simulink model "PGA_MPC_MODEL"  (R2024b)
settings: Solver=ode4  StartTime=0.0  StopTime=180  FixedStep=0.0005  RelTol=1e-3
values from neighbouring files (symbols this model uses):
  Road_Curvature_Map = [Global_S, Global_K]    [Road_Condition_Info.m]
  Road_Mu_Map = [Global_S, Global_Mu]    [Road_Condition_Info.m]
  Target_Speed_Map = [Global_S, Global_Vx]    [Road_Condition_Info.m]
undefined symbols (not defined in the file or in its folder): MotorData, Sim_Mu_Set, Sim_Vx_Set
libraries: Solver_SF x1
(part 3 of 3)

== matlab function PGA_MPC_MODEL/Subsystem1/MATLAB Function ==
  data: x_curr input; T_final_opt output; Solver_Status output; x_ref input; T_ref_upper_in input size=[4 1]; Vehicle_State input; Stiffness_Input input size=[2 1]; NN_Weights input; Constraints input; dt_in input; Mu_in input; Curv_in input; Delta_f_in input; Debug_Info output size=[5 1]
function [T_final_opt, Solver_Status, Debug_Info] = Lower_Layer_MPC_Fixed(...
x_curr, x_ref, T_ref_upper_in, Vehicle_State, Stiffness_Input, ...
NN_Weights, Constraints,dt_in, Mu_in, Curv_in, Delta_f_in) 
%#codegen
% =========================================================================
% 下层 MPC v44.0 (纯净执行者版：剔除所有底层干预规则，100% 权力移交 AI)
% =========================================================================
%% 0. 强制初始化
T_final_opt = zeros(4, 1, 'double');
Solver_Status = 0.0;
Debug_Info = zeros(5, 1, 'double');

%% 1. 解析 Vehicle_State 与滤波
Veh_State = double(reshape(Vehicle_State, 6, 1)); 
Vx = max(Veh_State(1), 1.0); 
Fz_fl_raw = max(Veh_State(3), 1000.0); Fz_fr_raw = max(Veh_State(4), 1000.0);
Fz_rl_raw = max(Veh_State(5), 1000.0); Fz_rr_raw = max(Veh_State(6), 1000.0);
persistent u_prev is_initialized Fz_fl_f Fz_fr_f Fz_rl_f Fz_rr_f
if isempty(u_prev)
u_prev = zeros(4, 1); 
Fz_fl_f = Fz_fl_raw; Fz_fr_f = Fz_fr_raw;
Fz_rl_f = Fz_rl_raw; Fz_rr_f = Fz_rr_raw;
is_initialized = false; 
end
alpha_fz = 0.2; 
Fz_fl_f = (1 - alpha_fz) * Fz_fl_f + alpha_fz * Fz_fl_raw;
Fz_fr_f = (1 - alpha_fz) * Fz_fr_f + alpha_fz * Fz_fr_raw;
Fz_rl_f = (1 - alpha_fz) * Fz_rl_f + alpha_fz * Fz_rl_raw;
Fz_rr_f = (1 - alpha_fz) * Fz_rr_f + alpha_fz * Fz_rr_raw;
Fz_fl = Fz_fl_f; Fz_fr = Fz_fr_f; Fz_rl = Fz_rl_f; Fz_rr = Fz_rr_f;
Fz_total = Fz_fl + Fz_fr + Fz_rl + Fz_rr;
dt = double(dt_in(1)); if dt <= 0, dt = 0.01; end
beta_in = double(x_curr(1)); r_in = double(x_curr(2));
x_ref_safe = double(reshape(x_ref, 2, 1));
% ★ 增加低通滤波隔离上层可能的高频毛刺 ★
T_ref_upper_raw = double(reshape(T_ref_upper_in, 4, 1)); 
persistent T_ref_filtered
if isempty(T_ref_filtered), T_ref_filtered = zeros(4, 1); end
alpha_T = 0.15; 
T_ref_filtered = (1 - alpha_T) * T_ref_filtered + alpha_T * T_ref_upper_raw;
T_ref_upper = T_ref_filtered; 
T_total_req = sum(T_ref_upper); 
delta_f_rad = double(Delta_f_in(1)); 

%% 2. 计算危险度 (仅用于摩擦圆限幅，不再用于权重干预)
rho_real = abs(double(Curv_in(1))); 
if rho_real < 1e-4, rho_real = 1e-4; end
ay_req_feedforward = (Vx^2) * rho_real; 
mu_est = max(0.15, double(Mu_in(1))); 
ay_max = mu_est * 9.81;
kappa_dyn = min(ay_req_feedforward / ay_max, 0.98);

%% 3. 提取贝叶斯权重 (完全绝对信任 AI)
Weights = double(reshape(NN_Weights, 5, 1));
Q_beta = max(Weights(1), 10.0); 
Q_yaw = max(Weights(2), 10.0);
R_alloc = max(Weights(3), 1.0); 
R_rate_base = max(Weights(4), 10.0); 
R_rate_vec = R_rate_base * ones(4, 1); 
% 绝对执行 AI 给出的防滑权重！
W_slip_base = max(Weights(5), 0.1);
W_slip_vec = zeros(4, 1);
W_slip_vec(1) = W_slip_base * ((Fz_total / 4) / Fz_fl);
W_slip_vec(2) = W_slip_base * ((Fz_total / 4) / Fz_fr);
W_slip_vec(3) = W_slip_base * ((Fz_total / 4) / Fz_rl);
W_slip_vec(4) = W_slip_base * ((Fz_total / 4) / Fz_rr);
%% 4. 总转矩硬约束 (废除 Mode_Signal 的规则干预)
% ★ 强制写死为 500000，确保总需求不打折，底层再无借口！
W_sum = 20000.0; 
%% 5. 前角前馈 LTV 模型构建 
Cf = double(Stiffness_Input(1)); Cr = double(Stiffness_Input(2));
if Cf < 20000, Cf = Cf * 57.3; end; if Cr < 20000, Cr = Cr * 57.3; end
Np = 25; Nc = 2; nx = 2; nu = 4;
m = 1810; Iz = 2765; lf = 1.152; lr = 1.528;
Cr_safe = max(Cr, Cf * (lf / lr) * 0.85); 
a11 = -(Cf + Cr_safe) / (m * Vx); 
a12 = ((lr * Cr_safe - lf * Cf) / (m * Vx^2)) - 1;
a21 = (lr * Cr_safe - lf * Cf) / Iz; 
a22 = -(lf^2 * Cf + lr^2 * Cr_safe) / (Iz * Vx);
G_mz = (1.6 / (2 * 0.3)) / Iz; 
A = eye(nx) + [a11, a12; a21, a22] * dt; 
B_row2 = G_mz * [-1, 1, -1, 1] * dt; 
B = [zeros(1, 4); B_row2];
B_delta_cont = [ Cf / (m * Vx) ; (lf * Cf) / Iz ];
B_delta = B_delta_cont * dt; 
Phi = zeros(nx * Np, nx); Gamma = zeros(nx * Np, nu * Nc);
Gamma_delta = zeros(nx * Np, 1); 
A_pow = eye(nx);
for i = 1:Np
A_pow = A * A_pow; 
Phi((i - 1) * nx + 1 : i * nx, :) = A_pow;
if i == 1, Gamma_delta(1:nx, 1) = B_delta;
else, Gamma_delta((i - 1) * nx + 1 : i * nx, 1) = A * Gamma_delta((i - 2) * nx + 1 : (i - 1) * nx, 1) + B_delta; end
for j = 1:min(i, Nc)
if i == j, term = B; else, term = A^(i - j) * B; end
Gamma((i - 1) * nx + 1 : i * nx, (j - 1) * nu + 1 : j * nu) = term;
end
end
%% 6. 代价函数构造 
Q_bar = blkdiag(kron(eye(Np), diag([Q_beta; Q_yaw])));
H_stab = Gamma' * Q_bar * Gamma;
X_free = Phi * [beta_in; r_in] + Gamma_delta * delta_f_rad; 
Y_ref = repmat(x_ref_safe, Np, 1);
f_stab = (X_free - Y_ref)' * Q_bar * Gamma;
R_alloc_mat = diag(repmat(R_alloc * ones(nu,1), Nc, 1));
H_alloc = R_alloc_mat; U_ref_vec = repmat(T_ref_upper, Nc, 1); 
f_alloc = -U_ref_vec' * R_alloc_mat;
R_rate_diag = repmat(R_rate_vec, Nc, 1); R_w_mat = diag(R_rate_diag);
D = zeros(nu * Nc, nu * Nc);
for k = 1:Nc
rows = (k - 1) * nu + (1:nu); cols = (k - 1) * nu + (1:nu);
D(rows, cols) = eye(nu); if k > 1, D(rows, cols - nu) = -eye(nu); end
end
H_rate = D' * R_w_mat * D;
d0 = zeros(nu * Nc, 1); d0(1:nu) = u_prev; f_rate = -d0' * R_w_mat * D;
H_sum = zeros(nu * Nc, nu * Nc); f_sum = zeros(1, nu * Nc);
for k_step = 1:Nc
idx = (k_step - 1) * nu + (1:nu);
H_sum(idx, idx) = W_sum * ones(nu, nu); f_sum(idx) = -W_sum * T_total_req * ones(1, nu);
end
H_slip = diag(repmat(W_slip_vec, Nc, 1)); f_slip = zeros(1, nu * Nc); 
H = 2 * (H_stab + H_alloc + H_rate + H_sum + H_slip);
f = 2 * (f_stab + f_alloc + f_rate + f_sum + f_slip)'; 
H = (H + H') / 2 + 1e-6 * eye(size(H)); 
%% 7. 约束求解 (仅保留瞬态安全裕度包线 TSM，废除变化率动态干预)
Cons = double(Constraints);
T_motor_lim = max(min(abs(Cons(2)), 350), 0); 
Margin_TSM = 0.15; 
Effective_Limit = 1.0 - Margin_TSM; 
Friction_Capacity = sqrt(max(Effective_Limit^2 - kappa_dyn^2, 0.01));
Re = 0.347; 
T_dyn_max_fl = Fz_fl * mu_est * Friction_Capacity * Re;
T_dyn_max_fr = Fz_fr * mu_est * Friction_Capacity * Re;
T_dyn_max_rl = Fz_rl * mu_est * Friction_Capacity * Re;
T_dyn_max_rr = Fz_rr * mu_est * Friction_Capacity * Re;
ub_fl = min(T_dyn_max_fl, T_motor_lim); ub_fr = min(T_dyn_max_fr, T_motor_lim);
ub_rl = min(T_dyn_max_rl, T_motor_lim); ub_rr = min(T_dyn_max_rr, T_motor_lim);
ub0_base = [ub_fl; ub_fr; ub_rl; ub_rr]; lb0_base = -ub0_base; 
ub0 = repmat(ub0_base, Nc, 1); lb0 = repmat(lb0_base, Nc, 1);
% ★ 核心修复：废除基于 kappa 的 du_max 规则限幅！
% 让转矩平滑的任务 100% 移交给 AI 的 R_rate 权重！
du_max = 8000 * dt; % 允许的最大硬件物理变化率 (80Nm/step)
lb = lb0; ub = ub0;
for k = 1:nu
u_last = u_prev(k);
for step = 1:Nc
idx = (step - 1) * nu + k;
lb(idx) = max(lb(idx), u_last - du_max * step);
ub(idx) = min(ub(idx), u_last + du_max * step);
end
end
coder.extrinsic('quadprog'); coder.extrinsic('optimoptions');
options = optimoptions('quadprog', 'Display', 'off', 'Algorithm', 'interior-point-convex');
U0 = repmat(u_prev, Nc, 1); 
[U_mx, ~, flag_mx] = quadprog(H, f, [], [], [], [], lb, ub, U0, options);
flag = -1; if ~isempty(flag_mx), flag = double(flag_mx); end
U_native = zeros(nu * Nc, 1); if ~isempty(U_mx), U_native = double(U_mx); end
if flag > 0, T_out = U_native(1:4); Solver_Status = 1.0;
else, T_out = T_ref_upper; Solver_Status = -1.0; end
%% 8. 输出清洗与死区
for i = 1:4
if isnan(T_out(i)) || isinf(T_out(i)), T_out(i) = 0; 
elseif abs(T_out(i)) < 2.0, T_out(i) = 0; 
else, T_out(i) = max(min(T_out(i), 350), -350); end
end
u_prev = T_out; 
T_final_opt(:) = T_out; 
Debug_Info(:) = [Q_beta; R_alloc; R_rate_base; kappa_dyn; Solver_Status];
end
